simulink model "Simulacao"  (Simulink 8.2)
settings: Solver=ode4  SolverMode=SingleTasking  StartTime=0.0  StopTime=60  FixedStep=0.01  RelTol=1e-3
InitFcn:
  | PreLoad;
values from neighbouring files (symbols this model uses):
  A1 = [   0   1 ... (first row only)    [PreLoad.m]
  B = [B]    [PreLoad.m]
  C = [1 0; 0 1]    [PreLoad.m]
  D = zeros(size(C,1), size(B,2))    [PreLoad.m]
  T = 1    [PreLoad.m]
  xk0 = [300;40]    [PreLoad.m]
undefined symbols (not defined in the file): A, epsilon, R, rho, S, Umax
libraries: simulink x1
settings Model: Creator=Kawakami  LastModifiedBy=Eduardo
settings DataIOCC: LimitDataPoints=off  SaveOutput=off  SaveTime=off  TimeSaveName=t  SignalLoggingName=sigsOut
settings OptimizationCC: BooleanDataType=off
settings DebuggingCC: SaveWithParameterizedLinksMsg=none  SignalResolutionControl=TryResolveAllWithWarning  SolverPrmCheckMsg=none  MultiTaskDSMMsg=warning  MultiTaskCondExecSysMsg=none
settings HardwareCC: TargetUnknown=on
settings RTWCC: IncludeERTFirstTime=on

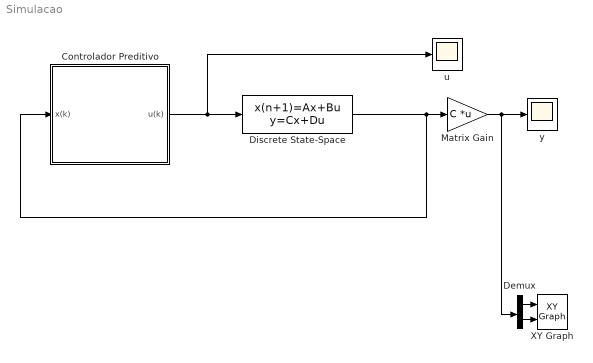
== system Simulacao ==
  "Controlador Preditivo  " : Subsystem  mask{A=A, B=B, S=S, R=R, Umax=Umax, T=T, rho=rho, epsilon=epsilon}
      mask prompts: A "Matriz Agregada A"; B "Matriz Agregada B"; S "S (custo quadrático)"; R "R (custo quadrático)"; Umax "Input Max"; T "T (passo da simulação)"; rho "rho (peso para o Gamma)"; epsilon "Epsilon (entra na matriz das igualdades)"
  Demux : Demux  Outputs=2
  Discrete State-Space : DiscreteStateSpace  A=A1  B=B  C=C  D=D  X0=xk0
  Matrix Gain : Gain  Gain=C  Multiplication=Matrix(K*u)  SaturateOnIntegerOverflow=on  OutDataTypeStr=Inherit: Same as input  ParamDataTypeStr=Inherit: Same as input
  XY Graph : simulink/Sinks/XY Graph  xmin=-300  xmax=300  ymin=-300  ymax=300  st=T
  u : Scope
      settings: TimeRange=10  YMin=-2  YMax=0.5
  y : Scope
      settings: TimeRange=10  YMin=-1  YMax=1  SaveName=ScopeData2
  wires:
  "Controlador Preditivo  "/1(u(k)) -> Discrete State-Space/1, u/1
  Discrete State-Space/1 -> "Controlador Preditivo  "/1(x(k)), Matrix Gain/1
  Matrix Gain/1 -> Demux/1, y/1
  Demux/2 -> XY Graph/2
  Demux/1 -> XY Graph/1

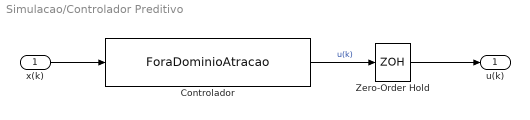
== system Simulacao/Controlador Preditivo   ==
  x(k) : Inport
  Controlador : S-Function  FunctionName=ForaDominioAtracao  Parameters=S, R, A, B, Umax, T, rho, epsilon  EnableBusSupport=off
  Zero-Order Hold : ZeroOrderHold  SampleTime=T
  u(k) : Outport
  wires:
  Zero-Order Hold/1 -> u(k)/1
  Controlador/1 -> Zero-Order Hold/1  "u(k)"
  x(k)/1 -> Controlador/1
